simulink model "SF009A_DutyCycThermProtn"  (R2013b)
settings: Solver=FixedStepDiscrete  SolverMode=SingleTasking  StartTime=0.0  StopTime=1  FixedStep=0.1  RelTol=1e-3
undefined symbols (not defined in the file): AbsltTThermLimCnt, ARCHGLBPRM_100MILLISEC_SEC_F32, CTRLRANDCUTFLT_CNT_U08, CTRLRTFLT_CNT_U08, CUTFLT_CNT_U08, DITHERMLIM_MOTNWTMTR_F32, DutyCycExcddCnt, DutyCycThermProtnAbsltCtrlTTblX, DutyCycThermProtnAbsltCtrlTTqTblY, DutyCycThermProtnAbsltCuTTblX, DutyCycThermProtnAbsltCuTTqTblY, DutyCycThermProtnAbsltMotVelBreakPt, DutyCycThermProtnAbsltTTqSlewHiLim, DutyCycThermProtnAbsltTTqSlewLoLim, DutyCycThermProtnCtrlT, DutyCycThermProtnCtrlTSeln, DutyCycThermProtnDutyCycFildThd, DutyCycThermProtnIgnOffCtrlEna, DutyCycThermProtnIgnOffMsgWaitTi, DutyCycThermProtnLstTblValNonStall, DutyCycThermProtnLstTblValStall, DutyCycThermProtnMotPrTSeln, DutyCycThermProtnMplr1NonStallTblY, DutyCycThermProtnMplr1StallTblY, DutyCycThermProtnMplr2NonStallTblY, DutyCycThermProtnMplr2StallTblY, DutyCycThermProtnMplr3NonStallTblY, DutyCycThermProtnMplr3StallTblY, DutyCycThermProtnMplr4NonStallTblY, DutyCycThermProtnMplr4StallTblY, DutyCycThermProtnMplr5NonStallTblY, DutyCycThermProtnMplr5StallTblY, DutyCycThermProtnMplr6NonStallTblY, DutyCycThermProtnMplr6StallTblY, DutyCycThermProtnMplrTblX, DutyCycThermProtnMplrTSeln, DutyCycThermProtnSlowFilTSeln, DutyCycThermProtnThermLoadLimTblX, DutyCycThermProtnThermLoadLimTblY, DutyCycThermProtnTqCmdSlewDwn, DutyCycThermProtnTqCmdSlewUp, FILVALMIN_ULS_F32, IGNTIOFFTHD_CNT_F32, NODEBSTEP_CNT_U16, NtcSts1, NvmGetErrSts1, ONEPERC_ULS_F32, TAU3_SEC_F32, TAU4_SEC_F32, TAU5_SEC_F32, TAU6_SEC_F32, THERMLOADLIMTBLIDX_ULS_U08
libraries: FixdToFloat x13, Fil x12, simulink x11, NxtrLim x10, NxtrMath x8, FloatToFixd x6, NxtrMax x6, NxtrMin x4, NxtrAbslt x2, NxtrNvM x1
(part 5 of 6)

== system SF009A_DutyCycThermProtn/DutyCycThermProtn/DutyCycThermProtnPer1/FiltSVReinit/VehTiVldEnabled/Filt3ExpDecay ==
  IgnTimeOffSel : Inport  RequirementInfo="{'linktype_rmi_doors' '0000a52a (/E-STEER Core/SubSystem Specifications/Application Functions/SF009A Thermal Duty Cycle Protection)' '#SF009A_285' 'true' 'REQ:  SF009A_285' '' } %GIDa_2f277cfa_04f7_4efd_8183_f26cc3ec11e8"
  FiltSVOrg : Inport  RequirementInfo="{'linktype_rmi_doors' '0000a52a (/E-STEER Core/SubSystem Specifications/Application Functions/SF009A Thermal Duty Cycle Protection)' '#SF009A_285' 'true' 'REQ:  SF009A_285' '' } %GIDa_6a80f34d_15bd_486f_9b83_6a28aa3fe0ad"  Port=2
  CopyRight2 : Subsystem  Description=|  mask(Copyright Information){none=on}
      | Copyright info block.                                               
      |                                                                     
      | Place copyright information at the top of every subsystem in design.
      mask prompts: none "No parameters"
      mask help: Place copyright information at the top of every subsystem in design.
      mask Display:
      | NxtrConf = 'Nexteer Confidential';
      | 
      | sys = bdroot; %handle for the current model ("system")
      | first = get_param(sys,'Created');
      | first = first(end-3:end);  %year is last four digits
      | 
      | last = get_param(sys,'LastModifiedDate');
      | if isempty(last)
      |     last = datestr(now,'yyyy');
      | else
      |     last = last(end-3:end);
      | end
      | 
      | if strcmp(first,last)
      |     fprintf('%s -- Copyright %s Nexteer',NxtrConf,first)
      | else
      |     fprintf('%s -- %s%s- %s Nexteer',NxtrConf,char(169),first,last)
      | end
  Exp_f32 : NxtrMath/Exp_f32  RequirementInfo="{'linktype_rmi_doors' '0000a52a (/E-STEER Core/SubSystem Specifications/Application Functions/SF009A Thermal Duty Cycle Protection)' '#SF009A_285' 'true' 'REQ:  SF009A_285' '' } %GIDa_b4229f1b_62cf_4fab_b7ac_5aae12ad4bab"  SFunctionSpec=single y1 = Exp_f32(single u1)  ShowSpec=on
      settings: AttributesFormatString=%<MaskType>
  Gain : Gain  RequirementInfo="{'linktype_rmi_doors' '0000a52a (/E-STEER Core/SubSystem Specifications/Application Functions/SF009A Thermal Duty Cycle Protection)' '#SF009A_285' 'true' 'REQ:  SF009A_285' '' } %GIDa_812109e6_0a0a_42eb_b926_01a1c9078124"  Gain=-1
  Product1 : Product  RequirementInfo="{'linktype_rmi_doors' '0000a52a (/E-STEER Core/SubSystem Specifications/Application Functions/SF009A Thermal Duty Cycle Protection)' '#SF009A_285' 'true' 'REQ:  SF009A_285' '' } %GIDa_513c209d_51b2_4ef5_92ed_fc68d3c652a9"  RndMeth=Zero
  Product2 : Product  RequirementInfo="{'linktype_rmi_doors' '0000a52a (/E-STEER Core/SubSystem Specifications/Application Functions/SF009A Thermal Duty Cycle Protection)' '#SF009A_285' 'true' 'REQ:  SF009A_285' '' } %GIDa_9ed37af2_4fbf_4a4c_9446_92cf6ee91099"  Inputs=*/  RndMeth=Zero
  Tau : Constant  RequirementInfo="{'linktype_rmi_doors' '0000a52a (/E-STEER Core/SubSystem Specifications/Application Functions/SF009A Thermal Duty Cycle Protection)' '#SF009A_285' 'true' 'REQ:  SF009A_285' '' } %GIDa_3ad883e5_7e2a_4b45_9df7_35a559f2c6ef"  Value=TAU3_SEC_F32
  FiltSV : Outport  RequirementInfo="{'linktype_rmi_doors' '0000a52a (/E-STEER Core/SubSystem Specifications/Application Functions/SF009A Thermal Duty Cycle Protection)' '#SF009A_285' 'true' 'REQ:  SF009A_285' '' } %GIDa_d206a6cd_498c_40ce_9958_2f76665f34bf"
  wires:
  FiltSVOrg/1 -> Product1/2
  Product1/1 -> FiltSV/1
  IgnTimeOffSel/1 -> Gain/1
  Tau/1 -> Product2/2
  Exp_f32/1 -> Product1/1
  Product2/1 -> Exp_f32/1
  Gain/1 -> Product2/1

== system SF009A_DutyCycThermProtn/DutyCycThermProtn/DutyCycThermProtnPer1/FiltSVReinit/VehTiVldEnabled/Filt4ExpDecay ==
  IgnTimeOffSel : Inport  RequirementInfo="{'linktype_rmi_doors' '0000a52a (/E-STEER Core/SubSystem Specifications/Application Functions/SF009A Thermal Duty Cycle Protection)' '#SF009A_285' 'true' 'REQ:  SF009A_285' '' } %GIDa_688e095e_1630_4ee3_972a_0461832cdda3"
  FiltSVOrg : Inport  RequirementInfo="{'linktype_rmi_doors' '0000a52a (/E-STEER Core/SubSystem Specifications/Application Functions/SF009A Thermal Duty Cycle Protection)' '#SF009A_285' 'true' 'REQ:  SF009A_285' '' } %GIDa_33abdde2_151f_4fc4_9a55_e2f8223019fd"  Port=2
  CopyRight2 : Subsystem  Description=|  mask(Copyright Information){none=on}
      | Copyright info block.                                               
      |                                                                     
      | Place copyright information at the top of every subsystem in design.
      mask prompts: none "No parameters"
      mask help: Place copyright information at the top of every subsystem in design.
      mask Display:
      | NxtrConf = 'Nexteer Confidential';
      | 
      | sys = bdroot; %handle for the current model ("system")
      | first = get_param(sys,'Created');
      | first = first(end-3:end);  %year is last four digits
      | 
      | last = get_param(sys,'LastModifiedDate');
      | if isempty(last)
      |     last = datestr(now,'yyyy');
      | else
      |     last = last(end-3:end);
      | end
      | 
      | if strcmp(first,last)
      |     fprintf('%s -- Copyright %s Nexteer',NxtrConf,first)
      | else
      |     fprintf('%s -- %s%s- %s Nexteer',NxtrConf,char(169),first,last)
      | end
  Exp_f32 : NxtrMath/Exp_f32  RequirementInfo="{'linktype_rmi_doors' '0000a52a (/E-STEER Core/SubSystem Specifications/Application Functions/SF009A Thermal Duty Cycle Protection)' '#SF009A_285' 'true' 'REQ:  SF009A_285' '' } %GIDa_9ab4e45b_1b1b_40ca_9537_5302fb2ce499"  SFunctionSpec=single y1 = Exp_f32(single u1)  ShowSpec=on
      settings: AttributesFormatString=%<MaskType>
  Gain : Gain  RequirementInfo="{'linktype_rmi_doors' '0000a52a (/E-STEER Core/SubSystem Specifications/Application Functions/SF009A Thermal Duty Cycle Protection)' '#SF009A_285' 'true' 'REQ:  SF009A_285' '' } %GIDa_ae4547df_6077_493c_bd57_9f901f4fd88e"  Gain=-1
  Product1 : Product  RequirementInfo="{'linktype_rmi_doors' '0000a52a (/E-STEER Core/SubSystem Specifications/Application Functions/SF009A Thermal Duty Cycle Protection)' '#SF009A_285' 'true' 'REQ:  SF009A_285' '' } %GIDa_0394ebf4_f70b_4d0f_9f33_5e25d2d33165"  RndMeth=Zero
  Product2 : Product  RequirementInfo="{'linktype_rmi_doors' '0000a52a (/E-STEER Core/SubSystem Specifications/Application Functions/SF009A Thermal Duty Cycle Protection)' '#SF009A_285' 'true' 'REQ:  SF009A_285' '' } %GIDa_031938eb_88a5_4562_96f1_5b0d01f7e7d0"  Inputs=*/  RndMeth=Zero
  Tau : Constant  RequirementInfo="{'linktype_rmi_doors' '0000a52a (/E-STEER Core/SubSystem Specifications/Application Functions/SF009A Thermal Duty Cycle Protection)' '#SF009A_285' 'true' 'REQ:  SF009A_285' '' } %GIDa_2afa65fd_4a07_43e0_808b_6dfeb622c5cf"  Value=TAU4_SEC_F32
  FiltSV : Outport  RequirementInfo="{'linktype_rmi_doors' '0000a52a (/E-STEER Core/SubSystem Specifications/Application Functions/SF009A Thermal Duty Cycle Protection)' '#SF009A_285' 'true' 'REQ:  SF009A_285' '' } %GIDa_09e81401_3187_40f5_b989_31a238aef27e"
  wires:
  FiltSVOrg/1 -> Product1/2
  Product1/1 -> FiltSV/1
  IgnTimeOffSel/1 -> Gain/1
  Tau/1 -> Product2/2
  Exp_f32/1 -> Product1/1
  Product2/1 -> Exp_f32/1
  Gain/1 -> Product2/1

== system SF009A_DutyCycThermProtn/DutyCycThermProtn/DutyCycThermProtnPer1/FiltSVReinit/VehTiVldEnabled/Filt5ExpDecay ==
  IgnTimeOffSel : Inport  RequirementInfo="{'linktype_rmi_doors' '0000a52a (/E-STEER Core/SubSystem Specifications/Application Functions/SF009A Thermal Duty Cycle Protection)' '#SF009A_285' 'true' 'REQ:  SF009A_285' '' } %GIDa_4b3c6625_036b_454a_a724_14ca2dcbb2da"
  FiltSVOrg : Inport  RequirementInfo="{'linktype_rmi_doors' '0000a52a (/E-STEER Core/SubSystem Specifications/Application Functions/SF009A Thermal Duty Cycle Protection)' '#SF009A_285' 'true' 'REQ:  SF009A_285' '' } %GIDa_6a4306e6_23dd_484c_b80e_68c6e3bc06b4"  Port=2
  CopyRight2 : Subsystem  Description=|  mask(Copyright Information){none=on}
      | Copyright info block.                                               
      |                                                                     
      | Place copyright information at the top of every subsystem in design.
      mask prompts: none "No parameters"
      mask help: Place copyright information at the top of every subsystem in design.
      mask Display:
      | NxtrConf = 'Nexteer Confidential';
      | 
      | sys = bdroot; %handle for the current model ("system")
      | first = get_param(sys,'Created');
      | first = first(end-3:end);  %year is last four digits
      | 
      | last = get_param(sys,'LastModifiedDate');
      | if isempty(last)
      |     last = datestr(now,'yyyy');
      | else
      |     last = last(end-3:end);
      | end
      | 
      | if strcmp(first,last)
      |     fprintf('%s -- Copyright %s Nexteer',NxtrConf,first)
      | else
      |     fprintf('%s -- %s%s- %s Nexteer',NxtrConf,char(169),first,last)
      | end
  Exp_f32 : NxtrMath/Exp_f32  RequirementInfo="{'linktype_rmi_doors' '0000a52a (/E-STEER Core/SubSystem Specifications/Application Functions/SF009A Thermal Duty Cycle Protection)' '#SF009A_285' 'true' 'REQ:  SF009A_285' '' } %GIDa_729f0013_7065_409d_b238_6136c9e3c98a"  SFunctionSpec=single y1 = Exp_f32(single u1)  ShowSpec=on
      settings: AttributesFormatString=%<MaskType>
  Gain : Gain  RequirementInfo="{'linktype_rmi_doors' '0000a52a (/E-STEER Core/SubSystem Specifications/Application Functions/SF009A Thermal Duty Cycle Protection)' '#SF009A_285' 'true' 'REQ:  SF009A_285' '' } %GIDa_bbcc1544_a7e8_4ae1_a20b_cd0ae4505034"  Gain=-1
  Product1 : Product  RequirementInfo="{'linktype_rmi_doors' '0000a52a (/E-STEER Core/SubSystem Specifications/Application Functions/SF009A Thermal Duty Cycle Protection)' '#SF009A_285' 'true' 'REQ:  SF009A_285' '' } %GIDa_be0cdc15_84dd_4bed_943b_4c704b26c2bc"  RndMeth=Zero
  Product2 : Product  RequirementInfo="{'linktype_rmi_doors' '0000a52a (/E-STEER Core/SubSystem Specifications/Application Functions/SF009A Thermal Duty Cycle Protection)' '#SF009A_285' 'true' 'REQ:  SF009A_285' '' } %GIDa_314f3b14_1b37_4b85_9ca8_b369e9216989"  Inputs=*/  RndMeth=Zero
  Tau : Constant  RequirementInfo="{'linktype_rmi_doors' '0000a52a (/E-STEER Core/SubSystem Specifications/Application Functions/SF009A Thermal Duty Cycle Protection)' '#SF009A_285' 'true' 'REQ:  SF009A_285' '' } %GIDa_d1fd6718_b6b6_439a_9b30_27e3c174fb58"  Value=TAU5_SEC_F32
  FiltSV : Outport  RequirementInfo="{'linktype_rmi_doors' '0000a52a (/E-STEER Core/SubSystem Specifications/Application Functions/SF009A Thermal Duty Cycle Protection)' '#SF009A_285' 'true' 'REQ:  SF009A_285' '' } %GIDa_b586d7b9_90b1_4c51_9dde_316f6a7aeae4"
  wires:
  FiltSVOrg/1 -> Product1/2
  Product1/1 -> FiltSV/1
  IgnTimeOffSel/1 -> Gain/1
  Tau/1 -> Product2/2
  Exp_f32/1 -> Product1/1
  Product2/1 -> Exp_f32/1
  Gain/1 -> Product2/1

== system SF009A_DutyCycThermProtn/DutyCycThermProtn/DutyCycThermProtnPer1/FiltSVReinit/VehTiVldEnabled/Filt6ExpDecay ==
  IgnTimeOffSel : Inport  RequirementInfo="{'linktype_rmi_doors' '0000a52a (/E-STEER Core/SubSystem Specifications/Application Functions/SF009A Thermal Duty Cycle Protection)' '#SF009A_285' 'true' 'REQ:  SF009A_285' '' } %GIDa_f5a9550d_806c_414d_8631_2d2380b76ab0"
  FiltSVOrg : Inport  RequirementInfo="{'linktype_rmi_doors' '0000a52a (/E-STEER Core/SubSystem Specifications/Application Functions/SF009A Thermal Duty Cycle Protection)' '#SF009A_285' 'true' 'REQ:  SF009A_285' '' } %GIDa_2defac87_6e02_413b_8475_9d4c2cb69c9e"  Port=2
  CopyRight2 : Subsystem  Description=|  mask(Copyright Information){none=on}
      | Copyright info block.                                               
      |                                                                     
      | Place copyright information at the top of every subsystem in design.
      mask prompts: none "No parameters"
      mask help: Place copyright information at the top of every subsystem in design.
      mask Display:
      | NxtrConf = 'Nexteer Confidential';
      | 
      | sys = bdroot; %handle for the current model ("system")
      | first = get_param(sys,'Created');
      | first = first(end-3:end);  %year is last four digits
      | 
      | last = get_param(sys,'LastModifiedDate');
      | if isempty(last)
      |     last = datestr(now,'yyyy');
      | else
      |     last = last(end-3:end);
      | end
      | 
      | if strcmp(first,last)
      |     fprintf('%s -- Copyright %s Nexteer',NxtrConf,first)
      | else
      |     fprintf('%s -- %s%s- %s Nexteer',NxtrConf,char(169),first,last)
      | end
  Exp_f32 : NxtrMath/Exp_f32  RequirementInfo="{'linktype_rmi_doors' '0000a52a (/E-STEER Core/SubSystem Specifications/Application Functions/SF009A Thermal Duty Cycle Protection)' '#SF009A_285' 'true' 'REQ:  SF009A_285' '' } %GIDa_4cd32e56_30f1_406e_b606_df838072ffb0"  SFunctionSpec=single y1 = Exp_f32(single u1)  ShowSpec=on
      settings: AttributesFormatString=%<MaskType>
  Gain : Gain  RequirementInfo="{'linktype_rmi_doors' '0000a52a (/E-STEER Core/SubSystem Specifications/Application Functions/SF009A Thermal Duty Cycle Protection)' '#SF009A_285' 'true' 'REQ:  SF009A_285' '' } %GIDa_db36424d_59ba_47c6_b149_da317fa6ea06"  Gain=-1
  Product1 : Product  RequirementInfo="{'linktype_rmi_doors' '0000a52a (/E-STEER Core/SubSystem Specifications/Application Functions/SF009A Thermal Duty Cycle Protection)' '#SF009A_285' 'true' 'REQ:  SF009A_285' '' } %GIDa_ddc8ce97_ddcc_41f8_8d8e_ba5cfb6ec71d"  RndMeth=Zero
  Product2 : Product  RequirementInfo="{'linktype_rmi_doors' '0000a52a (/E-STEER Core/SubSystem Specifications/Application Functions/SF009A Thermal Duty Cycle Protection)' '#SF009A_285' 'true' 'REQ:  SF009A_285' '' } %GIDa_ce23dae0_90a7_4b7e_89df_c3a4364a01fe"  Inputs=*/  RndMeth=Zero
  Tau : Constant  RequirementInfo="{'linktype_rmi_doors' '0000a52a (/E-STEER Core/SubSystem Specifications/Application Functions/SF009A Thermal Duty Cycle Protection)' '#SF009A_285' 'true' 'REQ:  SF009A_285' '' } %GIDa_9d922443_dae8_45b9_b8b2_6f88fda7eef6"  Value=TAU6_SEC_F32
  FiltSV : Outport  RequirementInfo="{'linktype_rmi_doors' '0000a52a (/E-STEER Core/SubSystem Specifications/Application Functions/SF009A Thermal Duty Cycle Protection)' '#SF009A_285' 'true' 'REQ:  SF009A_285' '' } %GIDa_e2442da6_9164_440b_b69a_c1998b02fa69"
  wires:
  FiltSVOrg/1 -> Product1/2
  Product1/1 -> FiltSV/1
  IgnTimeOffSel/1 -> Gain/1
  Tau/1 -> Product2/2
  Exp_f32/1 -> Product1/1
  Product2/1 -> Exp_f32/1
  Gain/1 -> Product2/1

== system SF009A_DutyCycThermProtn/DutyCycThermProtn/DutyCycThermProtnPer1/LoadLimiting/FilterPercMax/CopyRight2 ==

== system SF009A_DutyCycThermProtn/DutyCycThermProtn/DutyCycThermProtnPer1/LoadLimiting/FilterPercMax/DutyCycLevel_DutyCycThermProtnDisabled ==
  Action Port : ActionPort  ActionType=then
  CopyRight2 : Subsystem  Description=|  mask(Copyright Information){none=on}
      | Copyright info block.                                               
      |                                                                     
      | Place copyright information at the top of every subsystem in design.
      mask prompts: none "No parameters"
      mask help: Place copyright information at the top of every subsystem in design.
      mask Display:
      | NxtrConf = 'Nexteer Confidential';
      | 
      | sys = bdroot; %handle for the current model ("system")
      | first = get_param(sys,'Created');
      | first = first(end-3:end);  %year is last four digits
      | 
      | last = get_param(sys,'LastModifiedDate');
      | if isempty(last)
      |     last = datestr(now,'yyyy');
      | else
      |     last = last(end-3:end);
      | end
      | 
      | if strcmp(first,last)
      |     fprintf('%s -- Copyright %s Nexteer',NxtrConf,first)
      | else
      |     fprintf('%s -- %s%s- %s Nexteer',NxtrConf,char(169),first,last)
      | end
  D_DEFEATDUTYCYCLELEVEL_ULS : Constant  RequirementInfo="{'linktype_rmi_doors' '0000a52a (/E-STEER Core/SubSystem Specifications/Application Functions/SF009A Thermal Duty Cycle Protection)' '#SF009A_168' 'true' 'REQ:  SF009A_168' '' } %GIDa_cf1cd60c_14ff_436d_a874_5ee49fc952e4"  Value=0  OutDataTypeStr=Inherit: Inherit via back propagation
  DutyCycleLevel : Outport
  wires:
  D_DEFEATDUTYCYCLELEVEL_ULS/1 -> DutyCycleLevel/1

== system SF009A_DutyCycThermProtn/DutyCycThermProtn/DutyCycThermProtnPer1/LoadLimiting/FilterPercMax/DutyCycLevel_DutyCycThermProtnEnabled ==
  MaxSlowFilt : Inport
  Action Port : ActionPort  ActionType=else
  CopyRight2 : Subsystem  Description=|  mask(Copyright Information){none=on}
      | Copyright info block.                                               
      |                                                                     
      | Place copyright information at the top of every subsystem in design.
      mask prompts: none "No parameters"
      mask help: Place copyright information at the top of every subsystem in design.
      mask Display:
      | NxtrConf = 'Nexteer Confidential';
      | 
      | sys = bdroot; %handle for the current model ("system")
      | first = get_param(sys,'Created');
      | first = first(end-3:end);  %year is last four digits
      | 
      | last = get_param(sys,'LastModifiedDate');
      | if isempty(last)
      |     last = datestr(now,'yyyy');
      | else
      |     last = last(end-3:end);
      | end
      | 
      | if strcmp(first,last)
      |     fprintf('%s -- Copyright %s Nexteer',NxtrConf,first)
      | else
      |     fprintf('%s -- %s%s- %s Nexteer',NxtrConf,char(169),first,last)
      | end
  LimStat_f2 : NxtrLim/LimStat_f32  LoLim=single(0)  HiLim=FILOUTPLIM_ULS_F32
      settings: AttributesFormatString=Lower Limit: %<LoLim>\nUpper Limit: %<HiLim>
  DutyCycleLevel : Outport
  wires:
  LimStat_f2/1 -> DutyCycleLevel/1
  MaxSlowFilt/1 -> LimStat_f2/1

== system SF009A_DutyCycThermProtn/DutyCycThermProtn/DutyCycThermProtnPer1/LoadLimiting/Multiplier/CopyRight2 ==

== system SF009A_DutyCycThermProtn/DutyCycThermProtn/DutyCycThermProtnPer1/LoadLimiting/Multiplier/NonStallCondition ==
  note: Lookup table structure for all tables changed from interpolation to step change for each temperature range.
      | For input values less than the first calibrated X value, the first Y value shall be used, and for input values greater than the largest calibrated X value, the last Y value shall be used.
  note: Non-Stall Condition
  note: Lookup method : Use Input below
  note: Lookup method : Use Input below
  note: Lookup method : Use Input below
  note: Lookup method : Use Input below
  note: Lookup method : Use Input below
  note: Lookup method : Use Input below
  note: The Lookup method used for all the 6 tables below is  "Use Input below" meaning Finds the element in x nearest and below the current input.
      | The corresponding element in y is the output. If there is no element in x below thecurrent input, the block finds the nearest element.
  Mult12Temp : Inport  RequirementInfo="{'linktype_rmi_doors' '0000a52a (/E-STEER Core/SubSystem Specifications/Application Functions/SF009A Thermal Duty Cycle Protection)' '#SF009A_224' 'true' 'REQ:  SF009A_224' '' } %GIDa_15a3ec26_ae13_4a01_898e_d603e4d6290a"
  Mult36TempSlc : Inport  RequirementInfo="{'linktype_rmi_doors' '0000a52a (/E-STEER Core/SubSystem Specifications/Application Functions/SF009A Thermal Duty Cycle Protection)' '#SF009A_225' 'true' 'REQ:  SF009A_225' '' } %GIDa_709b3fc5_f20d_404f_aaf0_efd71be834f5"  Port=2
  Action Port : ActionPort  ActionType=then
  CopyRight2 : Subsystem  Description=|  mask(Copyright Information){none=on}
      | Copyright info block.                                               
      |                                                                     
      | Place copyright information at the top of every subsystem in design.
      mask prompts: none "No parameters"
      mask help: Place copyright information at the top of every subsystem in design.
      mask Display:
      | NxtrConf = 'Nexteer Confidential';
      | 
      | sys = bdroot; %handle for the current model ("system")
      | first = get_param(sys,'Created');
      | first = first(end-3:end);  %year is last four digits
      | 
      | last = get_param(sys,'LastModifiedDate');
      | if isempty(last)
      |     last = datestr(now,'yyyy');
      | else
      |     last = last(end-3:end);
      | end
      | 
      | if strcmp(first,last)
      |     fprintf('%s -- Copyright %s Nexteer',NxtrConf,first)
      | else
      |     fprintf('%s -- %s%s- %s Nexteer',NxtrConf,char(169),first,last)
      | end
  Multiplier 1 Non-Stall Condition Table Lookup : Lookup  RequirementInfo="{'linktype_rmi_doors' '0000a52a (/E-STEER Core/SubSystem Specifications/Application Functions/SF009A Thermal Duty Cycle Protection)' '#SF009A_220' 'true' 'REQ:  SF009A_220' '' ; 'linktype_rmi_doors' '0000a52a (/E-STEER Core/SubSystem Specifications/Application Functions/SF009A Thermal Duty Cycle Protection)' '#SF009A_222' 'true' 'REQ:  SF009A_222' '' } %GIDa_040cbf65_89fb_47d6_bf76_c5ba937961d0"  InputValues=DutyCycThermProtnMplrTblX  Table=DutyCycThermProtnMplr1NonStallTblY  LookUpMeth=Use Input Below  OutDataTypeStr=Inherit: Inherit via back propagation
      settings: AttributesFormatString=Output: %<Table>\nInput: %<InputValues>
  Multiplier 2 Non-Stall Condition Table Lookup : Lookup  RequirementInfo="{'linktype_rmi_doors' '0000a52a (/E-STEER Core/SubSystem Specifications/Application Functions/SF009A Thermal Duty Cycle Protection)' '#SF009A_220' 'true' 'REQ:  SF009A_220' '' ; 'linktype_rmi_doors' '0000a52a (/E-STEER Core/SubSystem Specifications/Application Functions/SF009A Thermal Duty Cycle Protection)' '#SF009A_222' 'true' 'REQ:  SF009A_222' '' } %GIDa_8042ba93_215d_4368_8d45_d97009916637"  InputValues=DutyCycThermProtnMplrTblX  Table=DutyCycThermProtnMplr2NonStallTblY  LookUpMeth=Use Input Below  OutDataTypeStr=Inherit: Inherit via back propagation
      settings: AttributesFormatString=Output: %<Table>\nInput: %<InputValues>
  Multiplier 3 Non-Stall Condition Table Lookup : Lookup  RequirementInfo="{'linktype_rmi_doors' '0000a52a (/E-STEER Core/SubSystem Specifications/Application Functions/SF009A Thermal Duty Cycle Protection)' '#SF009A_220' 'true' 'REQ:  SF009A_220' '' ; 'linktype_rmi_doors' '0000a52a (/E-STEER Core/SubSystem Specifications/Application Functions/SF009A Thermal Duty Cycle Protection)' '#SF009A_222' 'true' 'REQ:  SF009A_222' '' } %GIDa_e9474d90_bdb6_4f84_bb81_e8f0e810b760"  InputValues=DutyCycThermProtnMplrTblX  Table=DutyCycThermProtnMplr3NonStallTblY  LookUpMeth=Use Input Below  OutDataTypeStr=Inherit: Inherit via back propagation
      settings: AttributesFormatString=Output: %<Table>\nInput: %<InputValues>
  Multiplier 4 Non-Stall Condition Table Lookup : Lookup  RequirementInfo="{'linktype_rmi_doors' '0000a52a (/E-STEER Core/SubSystem Specifications/Application Functions/SF009A Thermal Duty Cycle Protection)' '#SF009A_220' 'true' 'REQ:  SF009A_220' '' ; 'linktype_rmi_doors' '0000a52a (/E-STEER Core/SubSystem Specifications/Application Functions/SF009A Thermal Duty Cycle Protection)' '#SF009A_222' 'true' 'REQ:  SF009A_222' '' } %GIDa_5ec721af_8ce5_4ecd_944d_bf56e967375f"  InputValues=DutyCycThermProtnMplrTblX  Table=DutyCycThermProtnMplr4NonStallTblY  LookUpMeth=Use Input Below  OutDataTypeStr=Inherit: Inherit via back propagation
      settings: AttributesFormatString=Output: %<Table>\nInput: %<InputValues>
  Multiplier 5 Non-Stall Condition Table Lookup : Lookup  RequirementInfo="{'linktype_rmi_doors' '0000a52a (/E-STEER Core/SubSystem Specifications/Application Functions/SF009A Thermal Duty Cycle Protection)' '#SF009A_220' 'true' 'REQ:  SF009A_220' '' ; 'linktype_rmi_doors' '0000a52a (/E-STEER Core/SubSystem Specifications/Application Functions/SF009A Thermal Duty Cycle Protection)' '#SF009A_222' 'true' 'REQ:  SF009A_222' '' } %GIDa_b08bc230_3876_4054_b57c_d6da79976698"  InputValues=DutyCycThermProtnMplrTblX  Table=DutyCycThermProtnMplr5NonStallTblY  LookUpMeth=Use Input Below  OutDataTypeStr=Inherit: Inherit via back propagation
      settings: AttributesFormatString=Output: %<Table>\nInput: %<InputValues>
  Multiplier 6 Non-Stall Condition Table Lookup : Lookup  RequirementInfo="{'linktype_rmi_doors' '0000a52a (/E-STEER Core/SubSystem Specifications/Application Functions/SF009A Thermal Duty Cycle Protection)' '#SF009A_220' 'true' 'REQ:  SF009A_220' '' ; 'linktype_rmi_doors' '0000a52a (/E-STEER Core/SubSystem Specifications/Application Functions/SF009A Thermal Duty Cycle Protection)' '#SF009A_222' 'true' 'REQ:  SF009A_222' '' } %GIDa_31c1cbb5_f611_4930_9dac_12f61a73d29b"  InputValues=DutyCycThermProtnMplrTblX  Table=DutyCycThermProtnMplr6NonStallTblY  LookUpMeth=Use Input Below  OutDataTypeStr=Inherit: Inherit via back propagation
      settings: AttributesFormatString=Output: %<Table>\nInput: %<InputValues>
  Mux : Mux  Inputs=6
  Mult : Outport
  wires:
  Multiplier 1 Non-Stall Condition Table Lookup/1 -> Mux/1
  Multiplier 2 Non-Stall Condition Table Lookup/1 -> Mux/2
  Mult36TempSlc/1 -> Multiplier 6 Non-Stall Condition Table Lookup/1, Multiplier 5 Non-Stall Condition Table Lookup/1, Multiplier 3 Non-Stall Condition Table Lookup/1, Multiplier 4 Non-Stall Condition Table Lookup/1
  Multiplier 3 Non-Stall Condition Table Lookup/1 -> Mux/3
  Multiplier 4 Non-Stall Condition Table Lookup/1 -> Mux/4
  Multiplier 5 Non-Stall Condition Table Lookup/1 -> Mux/5
  Multiplier 6 Non-Stall Condition Table Lookup/1 -> Mux/6
  Mult12Temp/1 -> Multiplier 2 Non-Stall Condition Table Lookup/1, Multiplier 1 Non-Stall Condition Table Lookup/1
  Mux/1 -> Mult/1

== system SF009A_DutyCycThermProtn/DutyCycThermProtn/DutyCycThermProtnPer1/LoadLimiting/Multiplier/SlowFilTSeln_Mult12Temp ==
  Mult12Temp : Inport
  Action Port : ActionPort  ActionType=then
  CopyRight2 : Subsystem  Description=|  mask(Copyright Information){none=on}
      | Copyright info block.                                               
      |                                                                     
      | Place copyright information at the top of every subsystem in design.
      mask prompts: none "No parameters"
      mask help: Place copyright information at the top of every subsystem in design.
      mask Display:
      | NxtrConf = 'Nexteer Confidential';
      | 
      | sys = bdroot; %handle for the current model ("system")
      | first = get_param(sys,'Created');
      | first = first(end-3:end);  %year is last four digits
      | 
      | last = get_param(sys,'LastModifiedDate');
      | if isempty(last)
      |     last = datestr(now,'yyyy');
      | else
      |     last = last(end-3:end);
      | end
      | 
      | if strcmp(first,last)
      |     fprintf('%s -- Copyright %s Nexteer',NxtrConf,first)
      | else
      |     fprintf('%s -- %s%s- %s Nexteer',NxtrConf,char(169),first,last)
      | end
  Mult36TempSlc : Outport
  wires:
  Mult12Temp/1 -> Mult36TempSlc/1

== system SF009A_DutyCycThermProtn/DutyCycThermProtn/DutyCycThermProtnPer1/LoadLimiting/Multiplier/SlowFilTSeln_Mult36Temp ==
  Mult36Temp : Inport
  Action Port : ActionPort  ActionType=else
  CopyRight2 : Subsystem  Description=|  mask(Copyright Information){none=on}
      | Copyright info block.                                               
      |                                                                     
      | Place copyright information at the top of every subsystem in design.
      mask prompts: none "No parameters"
      mask help: Place copyright information at the top of every subsystem in design.
      mask Display:
      | NxtrConf = 'Nexteer Confidential';
      | 
      | sys = bdroot; %handle for the current model ("system")
      | first = get_param(sys,'Created');
      | first = first(end-3:end);  %year is last four digits
      | 
      | last = get_param(sys,'LastModifiedDate');
      | if isempty(last)
      |     last = datestr(now,'yyyy');
      | else
      |     last = last(end-3:end);
      | end
      | 
      | if strcmp(first,last)
      |     fprintf('%s -- Copyright %s Nexteer',NxtrConf,first)
      | else
      |     fprintf('%s -- %s%s- %s Nexteer',NxtrConf,char(169),first,last)
      | end
  Mult36TempSlc : Outport
  wires:
  Mult36Temp/1 -> Mult36TempSlc/1

== system SF009A_DutyCycThermProtn/DutyCycThermProtn/DutyCycThermProtnPer1/LoadLimiting/Multiplier/StallCondition ==
  note: Lookup table structure for all tables changed from interpolation to step change for each temperature range.
      | For input values less than the first calibrated X value, the first Y value shall be used, and for input values greater than the largest calibrated X value, the last Y value shall be used.
  note: Stall Condition
  note: The Lookup method used for all the 6 tables below is  "Use Input below" meaning Finds the element in x nearest and below the current input.
      | The corresponding element in y is the output. If there is no element in x below thecurrent input, the block finds the nearest element.
  note: Lookup method : Use Input below
  note: Lookup method : Use Input below
  note: Lookup method : Use Input below
  note: Lookup method : Use Input below
  note: Lookup method : Use Input below
  note: Lookup method : Use Input below
  Mult12Temp : Inport  RequirementInfo="{'linktype_rmi_doors' '0000a52a (/E-STEER Core/SubSystem Specifications/Application Functions/SF009A Thermal Duty Cycle Protection)' '#SF009A_224' 'true' 'REQ:  SF009A_224' '' } %GIDa_9e736f64_5371_48c6_b29d_98d7a04e2700"
  Mult36TempSlc : Inport  RequirementInfo="{'linktype_rmi_doors' '0000a52a (/E-STEER Core/SubSystem Specifications/Application Functions/SF009A Thermal Duty Cycle Protection)' '#SF009A_225' 'true' 'REQ:  SF009A_225' '' } %GIDa_553df6a3_e81e_4199_bb36_62f8d0306279"  Port=2
  Action Port : ActionPort  ActionType=else
  CopyRight2 : Subsystem  Description=|  mask(Copyright Information){none=on}
      | Copyright info block.                                               
      |                                                                     
      | Place copyright information at the top of every subsystem in design.
      mask prompts: none "No parameters"
      mask help: Place copyright information at the top of every subsystem in design.
      mask Display:
      | NxtrConf = 'Nexteer Confidential';
      | 
      | sys = bdroot; %handle for the current model ("system")
      | first = get_param(sys,'Created');
      | first = first(end-3:end);  %year is last four digits
      | 
      | last = get_param(sys,'LastModifiedDate');
      | if isempty(last)
      |     last = datestr(now,'yyyy');
      | else
      |     last = last(end-3:end);
      | end
      | 
      | if strcmp(first,last)
      |     fprintf('%s -- Copyright %s Nexteer',NxtrConf,first)
      | else
      |     fprintf('%s -- %s%s- %s Nexteer',NxtrConf,char(169),first,last)
      | end
  Multiplier 1 Stall Condition Table Lookup : Lookup  RequirementInfo="{'linktype_rmi_doors' '0000a52a (/E-STEER Core/SubSystem Specifications/Application Functions/SF009A Thermal Duty Cycle Protection)' '#SF009A_221' 'true' 'REQ:  SF009A_221' '' ; 'linktype_rmi_doors' '0000a52a (/E-STEER Core/SubSystem Specifications/Application Functions/SF009A Thermal Duty Cycle Protection)' '#SF009A_222' 'true' 'REQ:  SF009A_222' '' } %GIDa_9fd8bddf_55f4_40c2_9de1_5afa276fb2ae"  InputValues=DutyCycThermProtnMplrTblX  Table=DutyCycThermProtnMplr1StallTblY  LookUpMeth=Use Input Below  OutDataTypeStr=Inherit: Inherit via back propagation
      settings: AttributesFormatString=Output: %<Table>\nInput: %<InputValues>
  Multiplier 2 Stall Condition Table Lookup : Lookup  RequirementInfo="{'linktype_rmi_doors' '0000a52a (/E-STEER Core/SubSystem Specifications/Application Functions/SF009A Thermal Duty Cycle Protection)' '#SF009A_221' 'true' 'REQ:  SF009A_221' '' ; 'linktype_rmi_doors' '0000a52a (/E-STEER Core/SubSystem Specifications/Application Functions/SF009A Thermal Duty Cycle Protection)' '#SF009A_222' 'true' 'REQ:  SF009A_222' '' } %GIDa_d13a61f9_bc55_4f9c_9c82_b67ebcc5711f"  InputValues=DutyCycThermProtnMplrTblX  Table=DutyCycThermProtnMplr2StallTblY  LookUpMeth=Use Input Below  OutDataTypeStr=Inherit: Inherit via back propagation
      settings: AttributesFormatString=Output: %<Table>\nInput: %<InputValues>
  Multiplier 3 Stall Condition Table Lookup : Lookup  RequirementInfo="{'linktype_rmi_doors' '0000a52a (/E-STEER Core/SubSystem Specifications/Application Functions/SF009A Thermal Duty Cycle Protection)' '#SF009A_221' 'true' 'REQ:  SF009A_221' '' ; 'linktype_rmi_doors' '0000a52a (/E-STEER Core/SubSystem Specifications/Application Functions/SF009A Thermal Duty Cycle Protection)' '#SF009A_222' 'true' 'REQ:  SF009A_222' '' } %GIDa_e78f92bd_c818_4426_875e_d4129946569a"  InputValues=DutyCycThermProtnMplrTblX  Table=DutyCycThermProtnMplr3StallTblY  LookUpMeth=Use Input Below  OutDataTypeStr=Inherit: Inherit via back propagation
      settings: AttributesFormatString=Output: %<Table>\nInput: %<InputValues>
  Multiplier 4 Stall Condition Table Lookup : Lookup  RequirementInfo="{'linktype_rmi_doors' '0000a52a (/E-STEER Core/SubSystem Specifications/Application Functions/SF009A Thermal Duty Cycle Protection)' '#SF009A_221' 'true' 'REQ:  SF009A_221' '' ; 'linktype_rmi_doors' '0000a52a (/E-STEER Core/SubSystem Specifications/Application Functions/SF009A Thermal Duty Cycle Protection)' '#SF009A_222' 'true' 'REQ:  SF009A_222' '' } %GIDa_54fd5508_1ae5_4eef_8010_89a382576046"  InputValues=DutyCycThermProtnMplrTblX  Table=DutyCycThermProtnMplr4StallTblY  LookUpMeth=Use Input Below  OutDataTypeStr=Inherit: Inherit via back propagation
      settings: AttributesFormatString=Output: %<Table>\nInput: %<InputValues>
  Multiplier 5 Stall Condition Table Lookup : Lookup  RequirementInfo="{'linktype_rmi_doors' '0000a52a (/E-STEER Core/SubSystem Specifications/Application Functions/SF009A Thermal Duty Cycle Protection)' '#SF009A_221' 'true' 'REQ:  SF009A_221' '' ; 'linktype_rmi_doors' '0000a52a (/E-STEER Core/SubSystem Specifications/Application Functions/SF009A Thermal Duty Cycle Protection)' '#SF009A_222' 'true' 'REQ:  SF009A_222' '' } %GIDa_564254f9_1620_4814_afcf_4fcd885d6474"  InputValues=DutyCycThermProtnMplrTblX  Table=DutyCycThermProtnMplr5StallTblY  LookUpMeth=Use Input Below  OutDataTypeStr=Inherit: Inherit via back propagation
      settings: AttributesFormatString=Output: %<Table>\nInput: %<InputValues>
  Multiplier 6 Stall Condition Table Lookup : Lookup  RequirementInfo="{'linktype_rmi_doors' '0000a52a (/E-STEER Core/SubSystem Specifications/Application Functions/SF009A Thermal Duty Cycle Protection)' '#SF009A_221' 'true' 'REQ:  SF009A_221' '' ; 'linktype_rmi_doors' '0000a52a (/E-STEER Core/SubSystem Specifications/Application Functions/SF009A Thermal Duty Cycle Protection)' '#SF009A_222' 'true' 'REQ:  SF009A_222' '' } %GIDa_199596d5_92a0_4d88_bfbd_ade09bff1f42"  InputValues=DutyCycThermProtnMplrTblX  Table=DutyCycThermProtnMplr6StallTblY  LookUpMeth=Use Input Below  OutDataTypeStr=Inherit: Inherit via back propagation
      settings: AttributesFormatString=Output: %<Table>\nInput: %<InputValues>
  Mux : Mux  Inputs=6
  Mult : Outport
  wires:
  Multiplier 1 Stall Condition Table Lookup/1 -> Mux/1
  Multiplier 4 Stall Condition Table Lookup/1 -> Mux/4
  Mult12Temp/1 -> Multiplier 1 Stall Condition Table Lookup/1, Multiplier 2 Stall Condition Table Lookup/1
  Mult36TempSlc/1 -> Multiplier 3 Stall Condition Table Lookup/1, Multiplier 4 Stall Condition Table Lookup/1, Multiplier 5 Stall Condition Table Lookup/1, Multiplier 6 Stall Condition Table Lookup/1
  Multiplier 2 Stall Condition Table Lookup/1 -> Mux/2
  Multiplier 5 Stall Condition Table Lookup/1 -> Mux/5
  Multiplier 6 Stall Condition Table Lookup/1 -> Mux/6
  Multiplier 3 Stall Condition Table Lookup/1 -> Mux/3
  Mux/1 -> Mult/1

== system SF009A_DutyCycThermProtn/DutyCycThermProtn/DutyCycThermProtnPer1/LoadLimiting/PowerOffTasks/CopyRight2 ==

== system SF009A_DutyCycThermProtn/DutyCycThermProtn/DutyCycThermProtnPer1/LoadLimiting/ThermalLoadLimit/CopyRight2 ==

== system SF009A_DutyCycThermProtn/DutyCycThermProtn/DutyCycThermProtnPer1/LoadLimiting/ThermalLoadLimit/DutyCycleLevel_LstTblValNonStall ==
  Action Port : ActionPort  ActionType=then
  Constant : Constant  RequirementInfo="{'linktype_rmi_doors' '0000a52a (/E-STEER Core/SubSystem Specifications/Application Functions/SF009A Thermal Duty Cycle Protection)' '#SF009A_237' 'true' 'REQ:  SF009A_237' '' } %GIDa_2bdb37b2_90de_4932_bdc4_6093f9667a46"  Value=DutyCycThermProtnLstTblValNonStall
  CopyRight2 : Subsystem  Description=|  mask(Copyright Information){none=on}
      | Copyright info block.                                               
      |                                                                     
      | Place copyright information at the top of every subsystem in design.
      mask prompts: none "No parameters"
      mask help: Place copyright information at the top of every subsystem in design.
      mask Display:
      | NxtrConf = 'Nexteer Confidential';
      | 
      | sys = bdroot; %handle for the current model ("system")
      | first = get_param(sys,'Created');
      | first = first(end-3:end);  %year is last four digits
      | 
      | last = get_param(sys,'LastModifiedDate');
      | if isempty(last)
      |     last = datestr(now,'yyyy');
      | else
      |     last = last(end-3:end);
      | end
      | 
      | if strcmp(first,last)
      |     fprintf('%s -- Copyright %s Nexteer',NxtrConf,first)
      | else
      |     fprintf('%s -- %s%s- %s Nexteer',NxtrConf,char(169),first,last)
      | end
  DutyCycleLevel : Outport
  wires:
  Constant/1 -> DutyCycleLevel/1

== system SF009A_DutyCycThermProtn/DutyCycThermProtn/DutyCycThermProtnPer1/LoadLimiting/ThermalLoadLimit/DutyCycleLevel_LstTblValStall ==
  Action Port : ActionPort  ActionType=else
  CopyRight2 : Subsystem  Description=|  mask(Copyright Information){none=on}
      | Copyright info block.                                               
      |                                                                     
      | Place copyright information at the top of every subsystem in design.
      mask prompts: none "No parameters"
      mask help: Place copyright information at the top of every subsystem in design.
      mask Display:
      | NxtrConf = 'Nexteer Confidential';
      | 
      | sys = bdroot; %handle for the current model ("system")
      | first = get_param(sys,'Created');
      | first = first(end-3:end);  %year is last four digits
      | 
      | last = get_param(sys,'LastModifiedDate');
      | if isempty(last)
      |     last = datestr(now,'yyyy');
      | else
      |     last = last(end-3:end);
      | end
      | 
      | if strcmp(first,last)
      |     fprintf('%s -- Copyright %s Nexteer',NxtrConf,first)
      | else
      |     fprintf('%s -- %s%s- %s Nexteer',NxtrConf,char(169),first,last)
      | end
  Thermal Load (Torque Command) Limit Table2 : Constant  RequirementInfo="{'linktype_rmi_doors' '0000a52a (/E-STEER Core/SubSystem Specifications/Application Functions/SF009A Thermal Duty Cycle Protection)' '#SF009A_238' 'true' 'REQ:  SF009A_238' '' } %GIDa_b4fdb058_87f9_43b9_9a91_a70718fca0fe"  Value=DutyCycThermProtnLstTblValStall
  DutyCycleLevel : Outport
  wires:
  Thermal Load (Torque Command) Limit Table2/1 -> DutyCycleLevel/1

== system SF009A_DutyCycThermProtn/DutyCycThermProtn/DutyCycThermProtnPer1/TemperatureSelection/MplrTSelnDisabled/CopyRight2 ==

== system SF009A_DutyCycThermProtn/DutyCycThermProtn/DutyCycThermProtnPer1/TemperatureSelection/MplrTSelnEnabled/CopyRight2 ==

== system SF009A_DutyCycThermProtn/DutyCycThermProtn/DutyCycThermProtnPer1/TemperatureSelection/Mult12T_DiagcStsLimdTPrfmncDisabled/CopyRight2 ==

== system SF009A_DutyCycThermProtn/DutyCycThermProtn/DutyCycThermProtnPer1/TemperatureSelection/Mult12T_DiagcStsLimdTPrfmncDisabled/CtrlTSelnDisabled ==
  MotFetT : Inport
  Action Port : ActionPort  ActionType=else
  CopyRight2 : Subsystem  Description=|  mask(Copyright Information){none=on}
      | Copyright info block.                                               
      |                                                                     
      | Place copyright information at the top of every subsystem in design.
      mask prompts: none "No parameters"
      mask help: Place copyright information at the top of every subsystem in design.
      mask Display:
      | NxtrConf = 'Nexteer Confidential';
      | 
      | sys = bdroot; %handle for the current model ("system")
      | first = get_param(sys,'Created');
      | first = first(end-3:end);  %year is last four digits
      | 
      | last = get_param(sys,'LastModifiedDate');
      | if isempty(last)
      |     last = datestr(now,'yyyy');
      | else
      |     last = last(end-3:end);
      | end
      | 
      | if strcmp(first,last)
      |     fprintf('%s -- Copyright %s Nexteer',NxtrConf,first)
      | else
      |     fprintf('%s -- %s%s- %s Nexteer',NxtrConf,char(169),first,last)
      | end
  Mult12 : Outport
  wires:
  MotFetT/1 -> Mult12/1

== system SF009A_DutyCycThermProtn/DutyCycThermProtn/DutyCycThermProtnPer1/TemperatureSelection/Mult12T_DiagcStsLimdTPrfmncDisabled/CtrlTSelnEnabled ==
  EcuTFild : Inport
  Action Port : ActionPort  ActionType=then
  CopyRight2 : Subsystem  Description=|  mask(Copyright Information){none=on}
      | Copyright info block.                                               
      |                                                                     
      | Place copyright information at the top of every subsystem in design.
      mask prompts: none "No parameters"
      mask help: Place copyright information at the top of every subsystem in design.
      mask Display:
      | NxtrConf = 'Nexteer Confidential';
      | 
      | sys = bdroot; %handle for the current model ("system")
      | first = get_param(sys,'Created');
      | first = first(end-3:end);  %year is last four digits
      | 
      | last = get_param(sys,'LastModifiedDate');
      | if isempty(last)
      |     last = datestr(now,'yyyy');
      | else
      |     last = last(end-3:end);
      | end
      | 
      | if strcmp(first,last)
      |     fprintf('%s -- Copyright %s Nexteer',NxtrConf,first)
      | else
      |     fprintf('%s -- %s%s- %s Nexteer',NxtrConf,char(169),first,last)
      | end
  Mult12 : Outport
  wires:
  EcuTFild/1 -> Mult12/1

== system SF009A_DutyCycThermProtn/DutyCycThermProtn/DutyCycThermProtnPer1/TemperatureSelection/Mult12T_DiagcStsLimdTPrfmncEnabled/CopyRight2 ==

== system SF009A_DutyCycThermProtn/DutyCycThermProtn/DutyCycThermProtnPer1/TemperatureSelection/Mult36T_DiagcStsLimdTPrfmncDisabled/CopyRight2 ==

== system SF009A_DutyCycThermProtn/DutyCycThermProtn/DutyCycThermProtnPer1/TemperatureSelection/Mult36T_DiagcStsLimdTPrfmncDisabled/MotPrTSelnDisabled ==
  MotWidgT : Inport
  Action Port : ActionPort  ActionType=else
  CopyRight2 : Subsystem  Description=|  mask(Copyright Information){none=on}
      | Copyright info block.                                               
      |                                                                     
      | Place copyright information at the top of every subsystem in design.
      mask prompts: none "No parameters"
      mask help: Place copyright information at the top of every subsystem in design.
      mask Display:
      | NxtrConf = 'Nexteer Confidential';
      | 
      | sys = bdroot; %handle for the current model ("system")
      | first = get_param(sys,'Created');
      | first = first(end-3:end);  %year is last four digits
      | 
      | last = get_param(sys,'LastModifiedDate');
      | if isempty(last)
      |     last = datestr(now,'yyyy');
      | else
      |     last = last(end-3:end);
      | end
      | 
      | if strcmp(first,last)
      |     fprintf('%s -- Copyright %s Nexteer',NxtrConf,first)
      | else
      |     fprintf('%s -- %s%s- %s Nexteer',NxtrConf,char(169),first,last)
      | end
  Mult36 : Outport
  wires:
  MotWidgT/1 -> Mult36/1

== system SF009A_DutyCycThermProtn/DutyCycThermProtn/DutyCycThermProtnPer1/TemperatureSelection/Mult36T_DiagcStsLimdTPrfmncDisabled/MotPrTSelnEnabled ==
  MotMagT : Inport
  Action Port : ActionPort  ActionType=then
  CopyRight2 : Subsystem  Description=|  mask(Copyright Information){none=on}
      | Copyright info block.                                               
      |                                                                     
      | Place copyright information at the top of every subsystem in design.
      mask prompts: none "No parameters"
      mask help: Place copyright information at the top of every subsystem in design.
      mask Display:
      | NxtrConf = 'Nexteer Confidential';
      | 
      | sys = bdroot; %handle for the current model ("system")
      | first = get_param(sys,'Created');
      | first = first(end-3:end);  %year is last four digits
      | 
      | last = get_param(sys,'LastModifiedDate');
      | if isempty(last)
      |     last = datestr(now,'yyyy');
      | else
      |     last = last(end-3:end);
      | end
      | 
      | if strcmp(first,last)
      |     fprintf('%s -- Copyright %s Nexteer',NxtrConf,first)
      | else
      |     fprintf('%s -- %s%s- %s Nexteer',NxtrConf,char(169),first,last)
      | end
  Mult36 : Outport
  wires:
  MotMagT/1 -> Mult36/1

== system SF009A_DutyCycThermProtn/DutyCycThermProtn/DutyCycThermProtnPer1/TemperatureSelection/Mult36T_DiagcStsLimdTPrfmncEnabled/CopyRight2 ==

== system SF009A_DutyCycThermProtn/DutyCycThermProtn/DutyCycThermProtnPer1/TempratureLimiting/SetCtrlrAndCuTFltNtc/CopyRight2 ==

== system SF009A_DutyCycThermProtn/DutyCycThermProtn/DutyCycThermProtnPer1/TempratureLimiting/SetCtrlrTFltNtc/CopyRight2 ==

== system SF009A_DutyCycThermProtn/DutyCycThermProtn/DutyCycThermProtnPer1/TempratureLimiting/SetCuTFltNtc/CopyRight2 ==

== system SF009A_DutyCycThermProtn/DutyCycThermProtn/DutyCycThermProtnPer1/TempratureLimiting/SetNtc/CopyRight2 ==
